simulink model "HW03_Tirel_Sim1"  (R2020b)
settings: Solver=VariableStepAuto  StartTime=0.0  StopTime=10  RelTol=1e-3
values from neighbouring files (symbols this model uses):
  C = [kt 0 0 0 ... (first row only)    [HW03_Tirel_Mat2.m]
libraries: cstblocks x1, pid_lib x1
settings Model: Creator=DELL  LastModifiedBy=DELL

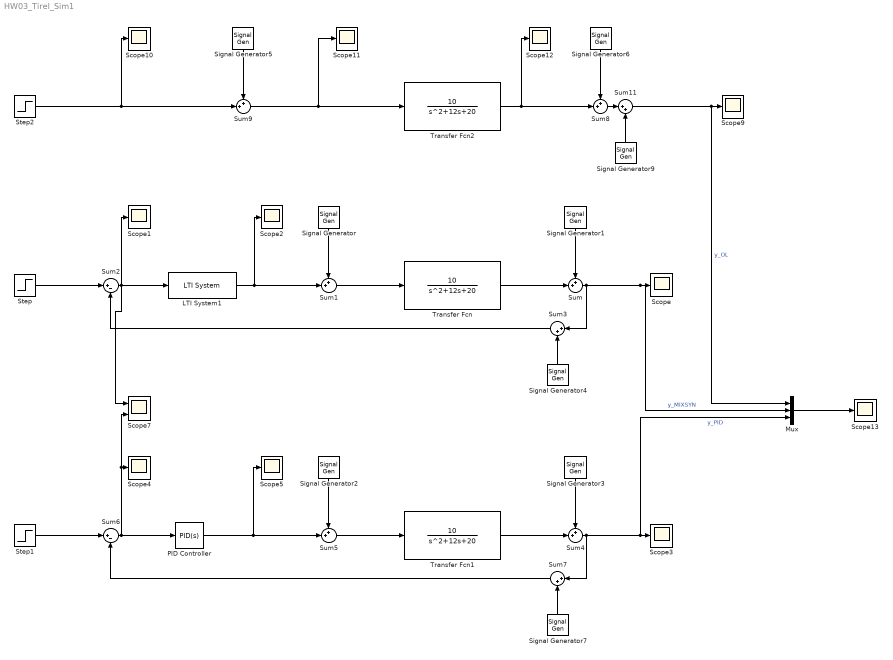
== system HW03_Tirel_Sim1 ==
  LTI System1 : cstblocks/LTI System  sys=tf(C)  IC=[]
  Mux : Mux  Inputs=3
  PID Controller : pid_lib/PID Controller  Controller=PID  Form=Parallel  TimeDomain=Continuous-time  UseExternalTs=off  SampleTime=-1  IntegratorMethod=Forward Euler  FilterMethod=Forward Euler  ControllerParametersSource=internal  P=3.64246622231547  I=10.2543715164682  D=0.191550186871053  UseFilter=on  N=37.1993217775763  TunerSelectOption=Transfer Function Based (PID Tuner App)  InitialConditionSource=internal  InitialConditionForIntegrator=0  InitialConditionForFilter=0  DifferentiatorICPrevScaledInput=0  ExternalReset=none  TrackingMode=off  Kt=1  LimitOutput=off  SatLimitsSource=internal  UpperSaturationLimit=inf  LowerSaturationLimit=-inf  LinearizeAsGain=on  AntiWindupMode=none  Kb=1  POutMin=[]  POutMax=[]  IOutMin=[]  IOutMax=[]  DOutMin=[]  DOutMax=[]  NOutMin=[]  NOutMax=[]  SumOutMin=[]  SumOutMax=[]  SaturationOutMin=[]  SaturationOutMax=[]  PParamMin=[]  PParamMax=[]  IParamMin=[]  IParamMax=[]  DParamMin=[]  DParamMax=[]  NParamMin=[]  NParamMax=[]  KbParamMin=[]  KbParamMax=[]  KtParamMin=[]  KtParamMax=[]  KbOutMin=[]  KbOutMax=[]  KtOutMin=[]  KtOutMax=[]  IntegratorOutMin=[]  IntegratorOutMax=[]  FilterOutMin=[]  FilterOutMax=[]  SumI1OutMin=[]  SumI1OutMax=[]  SumI2OutMin=[]  SumI2OutMax=[]  SumI3OutMin=[]  SumI3OutMax=[]  SumI4OutMin=[]  SumI4OutMax=[]  SumDOutMin=[]  SumDOutMax=[]  DifferentiatorOutMin=[]  DifferentiatorOutMax=[]  FilterDiffOutCoefMin=[]  FilterDiffOutCoefMax=[]  ReciprocalOutMin=[]  ReciprocalOutMax=[]  SumDenOutMin=[]  SumDenOutMax=[]  SumNumOutMin=[]  SumNumOutMax=[]  DivideOutMin=[]  DivideOutMax=[]  UdiffTsProdOutMin=[]  UdiffTsProdOutMax=[]  NTsProdOutMin=[]  NTsProdOutMax=[]  UintegralTsProdOutMin=[]  UintegralTsProdOutMax=[]  UngainTsProdOutMin=[]  UngainTsProdOutMax=[]  IntegratorContinuousStateAttributes=''  IntegratorStateMustResolveToSignalObject=off  IntegratorRTWStateStorageClass=Auto  FilterContinuousStateAttributes=''  FilterStateMustResolveToSignalObject=off  FilterRTWStateStorageClass=Auto  ParallelPVariant=InternalParameters  IdealPVariant=Disabled  IVariant=InternalParameters  DVariant=InternalParameters  IntegratorVariant=Continuous  SatVariant=Disabled  AWVariant=Passthrough  PCopyVariant=Disabled  TRVariant=Disabled  FdbkBlocksVariant=Forward  IdealPFdbkVariant=Disabled  SatFdbkVariant=Disabled  DerivativeFilterVariant=ContFilter  NVariant=InternalParameters  NCopyVariant=Disabled  FilterICVariant=InternalICsFilter  IntegratorICVariant=InternalICs  ExternalResetVariant=Disabled  TRSumVariant=Passthrough  SumFdbkVariant=Disabled  SumVariant=Sum_PID  TsampFilterVariant=InternalTs  TsampNgainVariant=Passthrough  TsampIntegralVariant=Passthrough  ExternalSaturationOutDataTypeStr=Inherit: Same as second input
  Scope{,1..5,9..13} (11 alike) : Scope
  Scope7 : Scope  NumInputPorts=2
  Signal Generator{,1..3,5..6} (6 alike) : SignalGenerator  Frequency=5  Units=rad/sec
  Signal Generator4 : SignalGenerator  Frequency=500  Units=rad/sec
  Signal Generator7 : SignalGenerator  Frequency=500  Units=rad/sec
  Signal Generator9 : SignalGenerator  Frequency=500  Units=rad/sec
  Step : Step  Time=0  After=10  SampleTime=0
  Step1 : Step  Time=0  After=10  SampleTime=0
  Step2 : Step  Time=0  After=10  SampleTime=0
  Sum{,1,4..5,8..9} (6 alike) : Sum  Inputs=++|
  Sum11 : Sum  Inputs=|++
  Sum2 : Sum  Inputs=|+-
  Sum3 : Sum  Inputs=|++
  Sum6 : Sum  Inputs=|+-
  Sum7 : Sum  Inputs=|++
  Transfer Fcn : TransferFcn  Numerator=[10]  Denominator=[1 12 20]
  Transfer Fcn1 : TransferFcn  Numerator=[10]  Denominator=[1 12 20]
  Transfer Fcn2 : TransferFcn  Numerator=[10]  Denominator=[1 12 20]
  wires:
  Transfer Fcn/1 -> Sum/2
  Sum/1 -> Sum3/1, Mux/2, Scope/1  "y_MIXSYN"
  Sum1/1 -> Transfer Fcn/1
  Step/1 -> Sum2/1
  Sum3/1 -> Sum2/2
  Sum6/1 -> PID Controller/1, Scope7/2, Scope4/1
  Sum5/1 -> Transfer Fcn1/1
  Sum7/1 -> Sum6/2
  Step1/1 -> Sum6/1
  Sum4/1 -> Sum7/1, Mux/3, Scope3/1  "y_PID"
  Transfer Fcn1/1 -> Sum4/2
  PID Controller/1 -> Scope5/1, Sum5/2
  Sum9/1 -> Scope11/1, Transfer Fcn2/1
  Transfer Fcn2/1 -> Scope12/1, Sum8/2
  Step2/1 -> Sum9/2, Scope10/1
  LTI System1/1 -> Scope2/1, Sum1/2
  Sum2/1 -> LTI System1/1, Scope1/1, Scope7/1
  Mux/1 -> Scope13/1
  Sum8/1 -> Sum11/1
  Sum11/1 -> Mux/1, Scope9/1  "y_OL"
  Signal Generator5/1 -> Sum9/1
  Signal Generator6/1 -> Sum8/1
  Signal Generator/1 -> Sum1/1
  Signal Generator1/1 -> Sum/1
  Signal Generator2/1 -> Sum5/1
  Signal Generator3/1 -> Sum4/1
  Signal Generator9/1 -> Sum11/2
  Signal Generator4/1 -> Sum3/2
  Signal Generator7/1 -> Sum7/2
